simulink model "prelab"  (R2022a)
settings: Solver=ode45  StartTime=0.0  StopTime=3  MaxStep=0.001  RelTol=1e-3
settings Model: Creator=zhong  LastModifiedBy=zhong

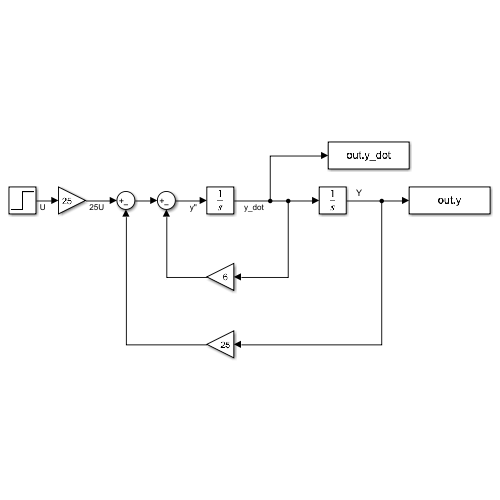
[thumbnail: Simulink's stored preview of the top-level diagram]
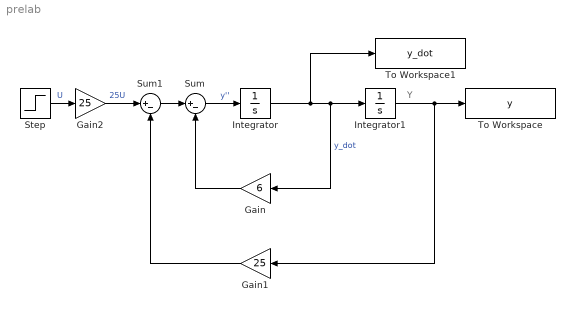
== system prelab ==
  note: Y
  Gain : Gain  Gain=6
  Gain1 : Gain  Gain=25
  Gain2 : Gain  Gain=25
  Integrator : Integrator
  Integrator1 : Integrator
  Step : Step  Time=0  SampleTime=0
  Sum : Sum  Inputs=|+-
  Sum1 : Sum  Inputs=|+-
  To Workspace : ToWorkspace  VariableName=y  SampleTime=-1
  To Workspace1 : ToWorkspace  VariableName=y_dot  SampleTime=-1
  wires:
  Sum/1 -> Integrator/1  "y''"
  Integrator/1 -> To Workspace1/1, Integrator1/1, Gain/1  "y_dot"
  Integrator1/1 -> Gain1/1, To Workspace/1
  Gain/1 -> Sum/2
  Sum1/1 -> Sum/1
  Step/1 -> Gain2/1  "U"
  Gain1/1 -> Sum1/2
  Gain2/1 -> Sum1/1  "25U"
